simulink model "tumbling_sim"  (R2018a)
settings: Solver=VariableStepAuto  StartTime=0.0  StopTime=5  MinStep=10e-13
values from neighbouring files (symbols this model uses):
  alpha = 0.5    [init_tumbling.m]
  gamma = 8    [init_tumbling.m]
  J = diag([Jxx Jyy Jzz])    [HTJHdet.m]    (also in init_tumbling.m = diag([1.3626 1.5333 0.3848]))
  q0 = [0.8034 0.1600 0.4272 0.3828]'    [init_tumbling.m]
  qd0 = [0.0379 0.6999 -0.2503 -0.0927]'    [init_tumbling.m]
settings Model: Creator=abinalexpothen  LastModifiedBy=abinalexpothen

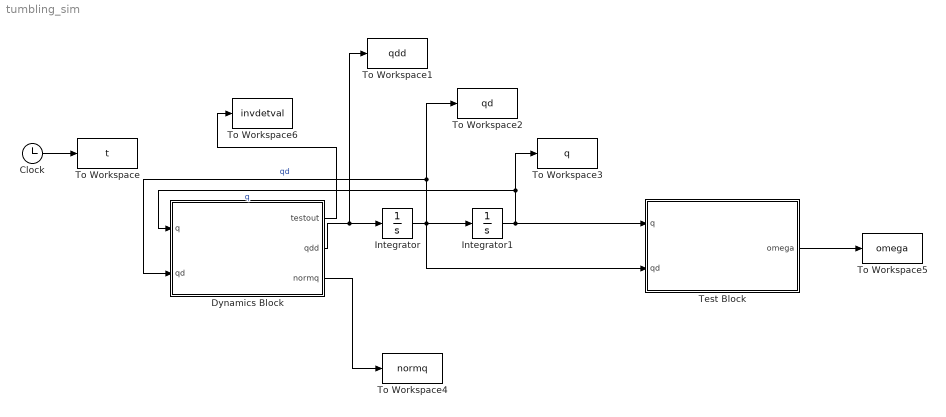
== system tumbling_sim ==
  Clock : Clock
  Dynamics Block : MATLAB Function  TreatAsAtomicUnit=on
  Integrator : Integrator  InitialCondition=qd0
  Integrator1 : Integrator  InitialCondition=q0
  Test Block : MATLAB Function  TreatAsAtomicUnit=on
  To Workspace : ToWorkspace  VariableName=t  SampleTime=-1
  To Workspace1 : ToWorkspace  VariableName=qdd  SampleTime=-1
  To Workspace2 : ToWorkspace  VariableName=qd  SampleTime=-1
  To Workspace3 : ToWorkspace  VariableName=q  SampleTime=-1
  To Workspace4 : ToWorkspace  VariableName=normq  SampleTime=-1
  To Workspace5 : ToWorkspace  VariableName=omega  SampleTime=-1
  To Workspace6 : ToWorkspace  VariableName=invdetval  SampleTime=-1
  wires:
  Dynamics Block/2(qdd) -> To Workspace1/1, Integrator/1
  Integrator/1 -> Dynamics Block/2(qd), To Workspace2/1, Test Block/2(qd), Integrator1/1  "qd"
  Integrator1/1 -> Test Block/1(q), Dynamics Block/1(q), To Workspace3/1  "q"
  Clock/1 -> To Workspace/1
  Dynamics Block/3(normq) -> To Workspace4/1
  Test Block/1(omega) -> To Workspace5/1
  Dynamics Block/1(testout) -> To Workspace6/1

== matlab function tumbling_sim/Test Block ==
  data: q input; omega output; qd input
function omega = testfun(q,qd)

H = 2*[-q(2) q(1) q(4) -q(3);
       -q(3) -q(4) q(1) q(2);
       -q(4) q(3) -q(2) q(1)];

omega = H*qd;

== matlab function tumbling_sim/Dynamics Block ==
  data: testout output; q input; qdd output; qd input; J parameter; normq output; alpha parameter; gamma parameter
function [testout, qdd, normq] = tumbling_dynamics(q,qd,J,alpha, gamma)

% modeling constraint functions
Am = 2*q';
bm = gamma-2*(qd')*qd-2*alpha*(q')*qd-gamma*(q')*q;

H = 2*[-q(2) q(1) q(4) -q(3);
       -q(3) -q(4) q(1) q(2);
       -q(4) q(3) -q(2) q(1)];

Hdot = 2*[-qd(2) qd(1) qd(4) -qd(3);
       -qd(3) -qd(4) qd(1) qd(2);
       -qd(4) qd(3) -qd(2) qd(1)];

qdd_u = -0.5*(H'*J* H)\(H'*H*Hdot'*J*H*qd);

qdd = qdd_u + (H'*J*H)^(-1)*(Am')*pinv(Am*(H'*J*H)^(-1)*Am')^(-1)*(bm-Am*qdd_u);
testout = det(H'*J* H);
normq = norm(q);
